simulink model "sim_mov"  (R2024a)
settings: Solver=VariableStepAuto  StartTime=0.0  StopTime=10.0  RelTol=1e-3
InitFcn:
  | m1=290;
  | b1=1000;
  | m2=59;
  | k1=16182;
  | k2=19000;
settings Model: Creator=ximen

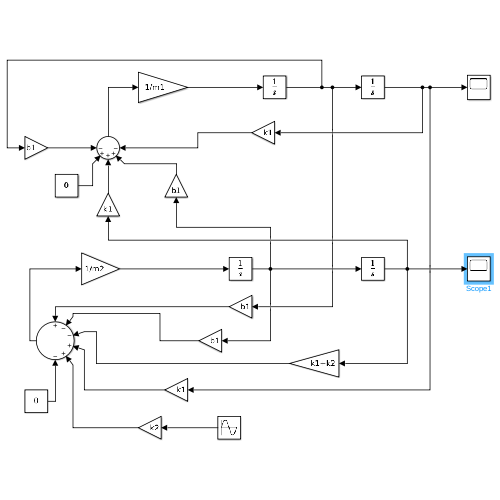
[thumbnail: Simulink's stored preview of the top-level diagram]
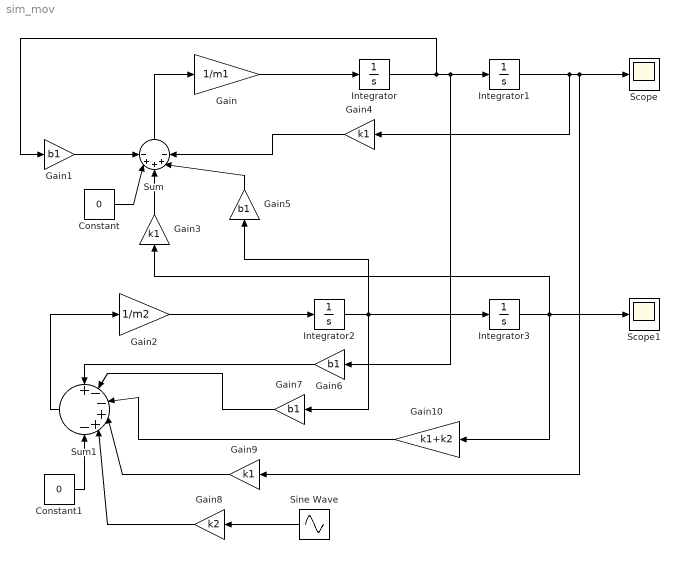
== system sim_mov ==
  Constant : Constant  Value=0
  Constant1 : Constant  Value=0
  Gain : Gain  Gain=1/m1
  Gain{1,5..7} (4 alike) : Gain  Gain=b1
  Gain10 : Gain  Gain=k1+k2
  Gain2 : Gain  Gain=1/m2
  Gain3 : Gain  Gain=k1
  Gain4 : Gain  Gain=k1
  Gain8 : Gain  Gain=k2
  Gain9 : Gain  Gain=k1
  Integrator{,1..3} (4 alike) : Integrator
  Scope : Scope
  Scope1 : Scope
  Sine Wave : Sin  Amplitude=0.05  Frequency=20*pi  SampleTime=0
  Sum : Sum  Inputs=-+++-
  Sum1 : Sum  Inputs=+--++-
  wires:
  Gain/1 -> Integrator/1
  Integrator1/1 -> Gain4/1, Gain9/1, Scope/1
  Integrator3/1 -> Gain10/1, Scope1/1, Gain3/1
  Integrator2/1 -> Gain7/1, Integrator3/1, Gain5/1
  Gain2/1 -> Integrator2/1
  Sum/1 -> Gain/1
  Gain1/1 -> Sum/1
  Gain3/1 -> Sum/3
  Constant/1 -> Sum/2
  Gain4/1 -> Sum/5
  Gain5/1 -> Sum/4
  Sum1/1 -> Gain2/1
  Gain6/1 -> Sum1/1
  Integrator/1 -> Gain1/1, Integrator1/1, Gain6/1
  Sine Wave/1 -> Gain8/1
  Gain7/1 -> Sum1/2
  Constant1/1 -> Sum1/6
  Gain8/1 -> Sum1/5
  Gain9/1 -> Sum1/4
  Gain10/1 -> Sum1/3
